simulink model "CM010C_GmG2kcaMcuCfg"  (R2013b)
settings: Solver=FixedStepDiscrete  SolverMode=SingleTasking  StartTime=0.0  StopTime=1  FixedStep=0.0005  RelTol=1e-3
values from neighbouring files (symbols this model uses):
  BATTVLTGSCAGFAC_ULS_F32 = DataDict.Constant    [CM010C_GmG2kcaMcuCfg_DataDict.m]
  BATTVLTGSWD1SCAGFAC_ULS_F32 = DataDict.Constant    [CM010C_GmG2kcaMcuCfg_DataDict.m]
undefined symbols (not defined in the file or in its folder): sigbuilder_block
libraries: CM010C_GmG2kcaMcuCfg_ModelLibrary x48, simulink x32
(part 2 of 2)

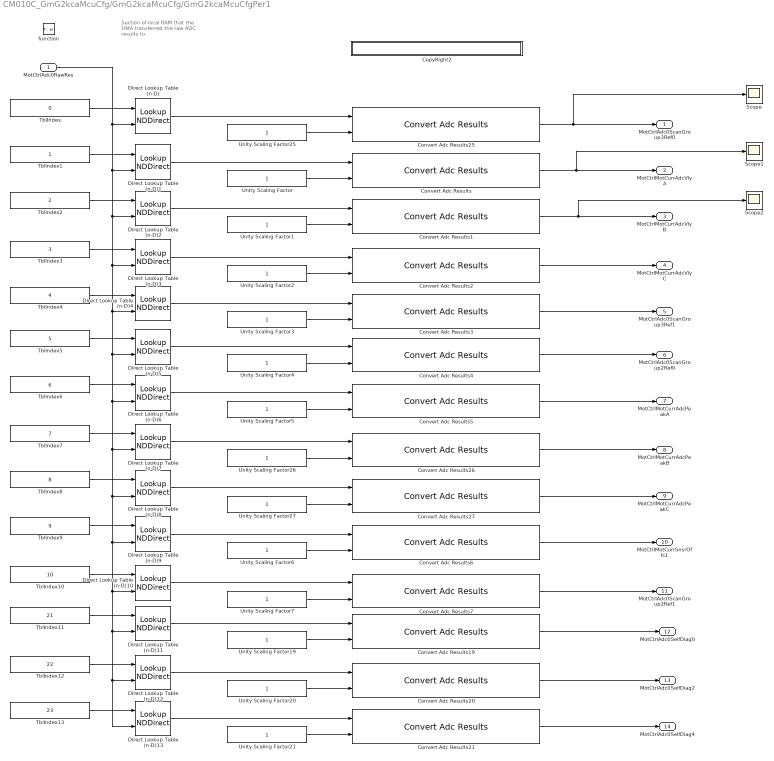
== system CM010C_GmG2kcaMcuCfg/GmG2kcaMcuCfg/GmG2kcaMcuCfgPer1 ==
  note: Section of local RAM that the
      | DMA transferred the raw
      | ADC results to
  MotCtrlAdc0RawRes : Inport
  function : TriggerPort  TriggerType=function-call
  Convert Adc Results{,1..7,19..21,25..27} (14 alike) : CM010C_GmG2kcaMcuCfg_ModelLibrary/Convert Adc Results
  CopyRight2 : Subsystem  Description=|  mask(Copyright Information){none=on}
      | Copyright info block.                                               
      |                                                                     
      | Place copyright information at the top of every subsystem in design.
      mask prompts: none "No parameters"
      mask help: Place copyright information at the top of every subsystem in design.
      mask Display:
      | NxtrConf = 'Nexteer Confidential';
      | 
      | sys = bdroot; %handle for the current model ("system")
      | first = get_param(sys,'Created');
      | first = first(end-3:end);  %year is last four digits
      | 
      | last = get_param(sys,'LastModifiedDate');
      | if isempty(last)
      |     last = datestr(now,'yyyy');
      | else
      |     last = last(end-3:end);
      | end
      | 
      | if strcmp(first,last)
      |     fprintf('%s -- Copyright %s Nexteer',NxtrConf,first)
      | else
      |     fprintf('%s -- %s%s- %s Nexteer',NxtrConf,char(169),first,last)
      | end
  Direct Lookup Table (n-D){,1..13} (14 alike) : LookupNDDirect  NumberOfTableDimensions=1  TableIsInput=on
  Scope : Scope
  Scope1 : Scope
  Scope2 : Scope
      settings: SaveName=ScopeData2
  TblIndex : Constant  Value=0  OutDataTypeStr=Inherit: Inherit via back propagation
  TblIndex1 : Constant  OutDataTypeStr=Inherit: Inherit via back propagation
  TblIndex10 : Constant  Value=10  OutDataTypeStr=Inherit: Inherit via back propagation
  TblIndex11 : Constant  Value=21  OutDataTypeStr=Inherit: Inherit via back propagation
  TblIndex12 : Constant  Value=22  OutDataTypeStr=Inherit: Inherit via back propagation
  TblIndex13 : Constant  Value=23  OutDataTypeStr=Inherit: Inherit via back propagation
  TblIndex2 : Constant  Value=2  OutDataTypeStr=Inherit: Inherit via back propagation
  TblIndex3 : Constant  Value=3  OutDataTypeStr=Inherit: Inherit via back propagation
  TblIndex4 : Constant  Value=4  OutDataTypeStr=Inherit: Inherit via back propagation
  TblIndex5 : Constant  Value=5  OutDataTypeStr=Inherit: Inherit via back propagation
  TblIndex6 : Constant  Value=6  OutDataTypeStr=Inherit: Inherit via back propagation
  TblIndex7 : Constant  Value=7  OutDataTypeStr=Inherit: Inherit via back propagation
  TblIndex8 : Constant  Value=8  OutDataTypeStr=Inherit: Inherit via back propagation
  TblIndex9 : Constant  Value=9  OutDataTypeStr=Inherit: Inherit via back propagation
  Unity Scaling Factor{,1..7,19..21,25..27} (14 alike) : Constant  OutDataTypeStr=single
  MotCtrlAdc0ScanGroup3Ref0 : Outport
  MotCtrlMotCurrAdcVlyA : Outport  Port=2
  MotCtrlMotCurrAdcVlyB : Outport  Port=3
  MotCtrlMotCurrAdcVlyC : Outport  Port=4
  MotCtrlAdc0ScanGroup3Ref1 : Outport  Port=5
  MotCtrlAdc0ScanGroup2Ref0 : Outport  Port=6
  MotCtrlMotCurrAdcPeakA : Outport  Port=7
  MotCtrlMotCurrAdcPeakB : Outport  Port=8
  MotCtrlMotCurrAdcPeakC : Outport  Port=9
  MotCtrlMotCurrSnsrOffs1 : Outport  Port=10
  MotCtrlAdc0ScanGroup2Ref1 : Outport  Port=11
  MotCtrlAdc0SelfDiag0 : Outport  Port=12
  MotCtrlAdc0SelfDiag2 : Outport  Port=13
  MotCtrlAdc0SelfDiag4 : Outport  Port=14
  wires:
  Unity Scaling Factor/1 -> Convert Adc Results/2
  Unity Scaling Factor1/1 -> Convert Adc Results1/2
  Unity Scaling Factor2/1 -> Convert Adc Results2/2
  Unity Scaling Factor3/1 -> Convert Adc Results3/2
  Unity Scaling Factor4/1 -> Convert Adc Results4/2
  Unity Scaling Factor5/1 -> Convert Adc Results5/2
  Unity Scaling Factor6/1 -> Convert Adc Results6/2
  Unity Scaling Factor7/1 -> Convert Adc Results7/2
  Unity Scaling Factor19/1 -> Convert Adc Results19/2
  Unity Scaling Factor20/1 -> Convert Adc Results20/2
  Direct Lookup Table (n-D)/1 -> Convert Adc Results25/1
  Unity Scaling Factor21/1 -> Convert Adc Results21/2
  Convert Adc Results2/1 -> MotCtrlMotCurrAdcVlyC/1
  Convert Adc Results19/1 -> MotCtrlAdc0SelfDiag0/1
  Convert Adc Results20/1 -> MotCtrlAdc0SelfDiag2/1
  Convert Adc Results21/1 -> MotCtrlAdc0SelfDiag4/1
  Unity Scaling Factor25/1 -> Convert Adc Results25/2
  Unity Scaling Factor26/1 -> Convert Adc Results26/2
  Unity Scaling Factor27/1 -> Convert Adc Results27/2
  Convert Adc Results1/1 -> Scope2/1, MotCtrlMotCurrAdcVlyB/1
  Convert Adc Results/1 -> Scope1/1, MotCtrlMotCurrAdcVlyA/1
  Convert Adc Results3/1 -> MotCtrlAdc0ScanGroup3Ref1/1
  Convert Adc Results4/1 -> MotCtrlAdc0ScanGroup2Ref0/1
  Convert Adc Results5/1 -> MotCtrlMotCurrAdcPeakA/1
  Convert Adc Results26/1 -> MotCtrlMotCurrAdcPeakB/1
  Convert Adc Results27/1 -> MotCtrlMotCurrAdcPeakC/1
  Convert Adc Results6/1 -> MotCtrlMotCurrSnsrOffs1/1
  Convert Adc Results7/1 -> MotCtrlAdc0ScanGroup2Ref1/1
  TblIndex/1 -> Direct Lookup Table (n-D)/1
  Convert Adc Results25/1 -> Scope/1, MotCtrlAdc0ScanGroup3Ref0/1
  TblIndex1/1 -> Direct Lookup Table (n-D)1/1
  TblIndex2/1 -> Direct Lookup Table (n-D)2/1
  Direct Lookup Table (n-D)1/1 -> Convert Adc Results/1
  Direct Lookup Table (n-D)2/1 -> Convert Adc Results1/1
  TblIndex3/1 -> Direct Lookup Table (n-D)3/1
  TblIndex4/1 -> Direct Lookup Table (n-D)4/1
  TblIndex5/1 -> Direct Lookup Table (n-D)5/1
  Direct Lookup Table (n-D)3/1 -> Convert Adc Results2/1
  Direct Lookup Table (n-D)4/1 -> Convert Adc Results3/1
  Direct Lookup Table (n-D)5/1 -> Convert Adc Results4/1
  TblIndex6/1 -> Direct Lookup Table (n-D)6/1
  TblIndex7/1 -> Direct Lookup Table (n-D)7/1
  TblIndex8/1 -> Direct Lookup Table (n-D)8/1
  TblIndex9/1 -> Direct Lookup Table (n-D)9/1
  TblIndex10/1 -> Direct Lookup Table (n-D)10/1
  TblIndex11/1 -> Direct Lookup Table (n-D)11/1
  Direct Lookup Table (n-D)6/1 -> Convert Adc Results5/1
  Direct Lookup Table (n-D)7/1 -> Convert Adc Results26/1
  Direct Lookup Table (n-D)8/1 -> Convert Adc Results27/1
  Direct Lookup Table (n-D)9/1 -> Convert Adc Results6/1
  Direct Lookup Table (n-D)10/1 -> Convert Adc Results7/1
  Direct Lookup Table (n-D)11/1 -> Convert Adc Results19/1
  TblIndex12/1 -> Direct Lookup Table (n-D)12/1
  MotCtrlAdc0RawRes/1 -> Direct Lookup Table (n-D)13/2, Direct Lookup Table (n-D)12/2, Direct Lookup Table (n-D)11/2, Direct Lookup Table (n-D)10/2, Direct Lookup Table (n-D)9/2, Direct Lookup Table (n-D)8/2, Direct Lookup Table (n-D)7/2, Direct Lookup Table (n-D)6/2, Direct Lookup Table (n-D)5/2, Direct Lookup Table (n-D)4/2, Direct Lookup Table (n-D)3/2, Direct Lookup Table (n-D)2/2, Direct Lookup Table (n-D)1/2, Direct Lookup Table (n-D)/2
  TblIndex13/1 -> Direct Lookup Table (n-D)13/1
  Direct Lookup Table (n-D)12/1 -> Convert Adc Results20/1
  Direct Lookup Table (n-D)13/1 -> Convert Adc Results21/1

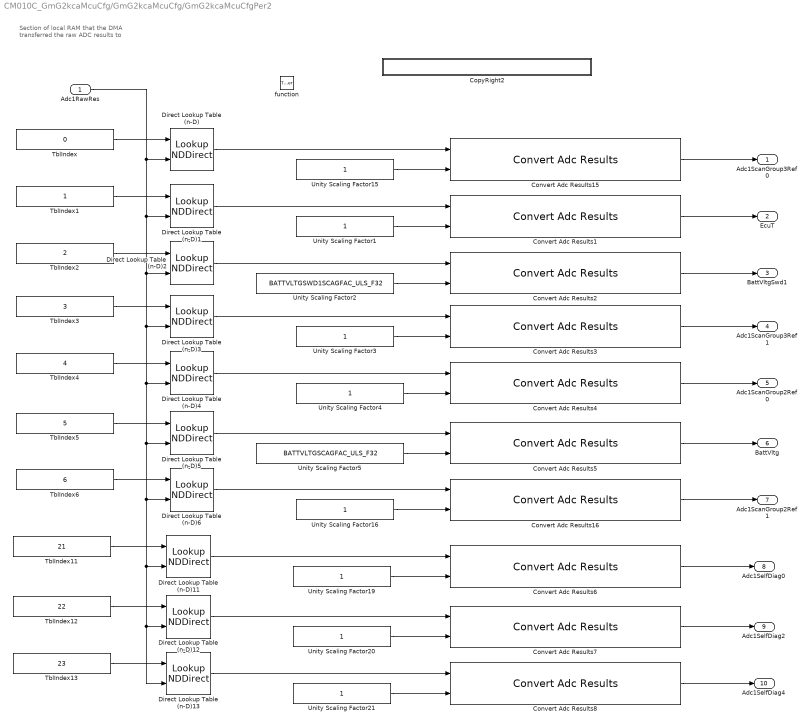
== system CM010C_GmG2kcaMcuCfg/GmG2kcaMcuCfg/GmG2kcaMcuCfgPer2 ==
  note: Section of local RAM that the
      | DMA transferred the raw
      | ADC results to
  Adc1RawRes : Inport
  function : TriggerPort  TriggerType=function-call
  Convert Adc Results{1..8,15..16} (10 alike) : CM010C_GmG2kcaMcuCfg_ModelLibrary/Convert Adc Results
  CopyRight2 : Subsystem  Description=|  mask(Copyright Information){none=on}
      | Copyright info block.                                               
      |                                                                     
      | Place copyright information at the top of every subsystem in design.
      mask prompts: none "No parameters"
      mask help: Place copyright information at the top of every subsystem in design.
      mask Display:
      | NxtrConf = 'Nexteer Confidential';
      | 
      | sys = bdroot; %handle for the current model ("system")
      | first = get_param(sys,'Created');
      | first = first(end-3:end);  %year is last four digits
      | 
      | last = get_param(sys,'LastModifiedDate');
      | if isempty(last)
      |     last = datestr(now,'yyyy');
      | else
      |     last = last(end-3:end);
      | end
      | 
      | if strcmp(first,last)
      |     fprintf('%s -- Copyright %s Nexteer',NxtrConf,first)
      | else
      |     fprintf('%s -- %s%s- %s Nexteer',NxtrConf,char(169),first,last)
      | end
  Direct Lookup Table (n-D){,1..6,11..13} (10 alike) : LookupNDDirect  NumberOfTableDimensions=1  TableIsInput=on
  TblIndex : Constant  Value=0  OutDataTypeStr=Inherit: Inherit via back propagation
  TblIndex1 : Constant  OutDataTypeStr=Inherit: Inherit via back propagation
  TblIndex11 : Constant  Value=21  OutDataTypeStr=Inherit: Inherit via back propagation
  TblIndex12 : Constant  Value=22  OutDataTypeStr=Inherit: Inherit via back propagation
  TblIndex13 : Constant  Value=23  OutDataTypeStr=Inherit: Inherit via back propagation
  TblIndex2 : Constant  Value=2  OutDataTypeStr=Inherit: Inherit via back propagation
  TblIndex3 : Constant  Value=3  OutDataTypeStr=Inherit: Inherit via back propagation
  TblIndex4 : Constant  Value=4  OutDataTypeStr=Inherit: Inherit via back propagation
  TblIndex5 : Constant  Value=5  OutDataTypeStr=Inherit: Inherit via back propagation
  TblIndex6 : Constant  Value=6  OutDataTypeStr=Inherit: Inherit via back propagation
  Unity Scaling Factor{1,3..4,15..16,19..21} (8 alike) : Constant  OutDataTypeStr=single
  Unity Scaling Factor2 : Constant  Value=BATTVLTGSWD1SCAGFAC_ULS_F32  OutDataTypeStr=single
  Unity Scaling Factor5 : Constant  Value=BATTVLTGSCAGFAC_ULS_F32  OutDataTypeStr=single
  Adc1ScanGroup3Ref0 : Outport
  EcuT : Outport  Port=2
  BattVltgSwd1 : Outport  Port=3
  Adc1ScanGroup3Ref1 : Outport  Port=4
  Adc1ScanGroup2Ref0 : Outport  Port=5
  BattVltg : Outport  Port=6
  Adc1ScanGroup2Ref1 : Outport  Port=7
  Adc1SelfDiag0 : Outport  Port=8
  Adc1SelfDiag2 : Outport  Port=9
  Adc1SelfDiag4 : Outport  Port=10
  wires:
  Convert Adc Results8/1 -> Adc1SelfDiag4/1
  Convert Adc Results7/1 -> Adc1SelfDiag2/1
  Convert Adc Results6/1 -> Adc1SelfDiag0/1
  Convert Adc Results1/1 -> EcuT/1
  Unity Scaling Factor21/1 -> Convert Adc Results8/2
  Direct Lookup Table (n-D)13/1 -> Convert Adc Results8/1
  Unity Scaling Factor20/1 -> Convert Adc Results7/2
  Direct Lookup Table (n-D)12/1 -> Convert Adc Results7/1
  Unity Scaling Factor19/1 -> Convert Adc Results6/2
  Direct Lookup Table (n-D)11/1 -> Convert Adc Results6/1
  Unity Scaling Factor5/1 -> Convert Adc Results5/2
  Unity Scaling Factor4/1 -> Convert Adc Results4/2
  Unity Scaling Factor3/1 -> Convert Adc Results3/2
  Unity Scaling Factor2/1 -> Convert Adc Results2/2
  Unity Scaling Factor1/1 -> Convert Adc Results1/2
  Unity Scaling Factor15/1 -> Convert Adc Results15/2
  Convert Adc Results15/1 -> Adc1ScanGroup3Ref0/1
  Unity Scaling Factor16/1 -> Convert Adc Results16/2
  Direct Lookup Table (n-D)/1 -> Convert Adc Results15/1
  Direct Lookup Table (n-D)1/1 -> Convert Adc Results1/1
  Direct Lookup Table (n-D)2/1 -> Convert Adc Results2/1
  Direct Lookup Table (n-D)3/1 -> Convert Adc Results3/1
  Direct Lookup Table (n-D)4/1 -> Convert Adc Results4/1
  Direct Lookup Table (n-D)5/1 -> Convert Adc Results5/1
  Direct Lookup Table (n-D)6/1 -> Convert Adc Results16/1
  Convert Adc Results2/1 -> BattVltgSwd1/1
  Convert Adc Results3/1 -> Adc1ScanGroup3Ref1/1
  Convert Adc Results4/1 -> Adc1ScanGroup2Ref0/1
  Convert Adc Results5/1 -> BattVltg/1
  Convert Adc Results16/1 -> Adc1ScanGroup2Ref1/1
  TblIndex/1 -> Direct Lookup Table (n-D)/1
  TblIndex1/1 -> Direct Lookup Table (n-D)1/1
  TblIndex2/1 -> Direct Lookup Table (n-D)2/1
  TblIndex3/1 -> Direct Lookup Table (n-D)3/1
  TblIndex4/1 -> Direct Lookup Table (n-D)4/1
  TblIndex5/1 -> Direct Lookup Table (n-D)5/1
  TblIndex6/1 -> Direct Lookup Table (n-D)6/1
  TblIndex11/1 -> Direct Lookup Table (n-D)11/1
  TblIndex12/1 -> Direct Lookup Table (n-D)12/1
  Adc1RawRes/1 -> Direct Lookup Table (n-D)/2, Direct Lookup Table (n-D)1/2, Direct Lookup Table (n-D)2/2, Direct Lookup Table (n-D)3/2, Direct Lookup Table (n-D)4/2, Direct Lookup Table (n-D)5/2, Direct Lookup Table (n-D)6/2, Direct Lookup Table (n-D)11/2, Direct Lookup Table (n-D)12/2, Direct Lookup Table (n-D)13/2
  TblIndex13/1 -> Direct Lookup Table (n-D)13/1

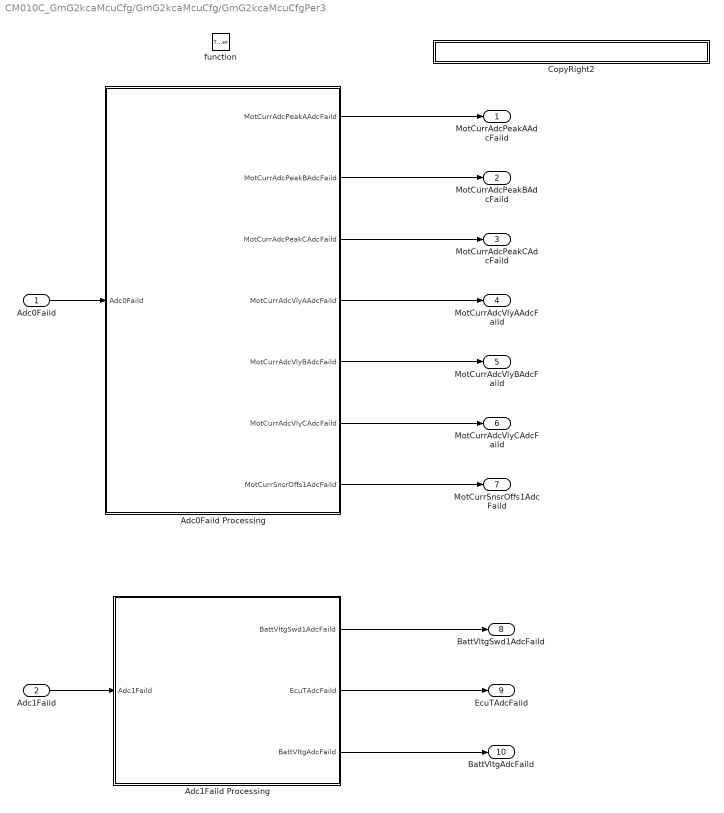
== system CM010C_GmG2kcaMcuCfg/GmG2kcaMcuCfg/GmG2kcaMcuCfgPer3 ==
  Adc0Faild : Inport
  Adc1Faild : Inport  Port=2
  function : TriggerPort  TriggerType=function-call
  Adc0Faild Processing : Subsystem  TreatAsAtomicUnit=on
  Adc1Faild Processing : Subsystem  TreatAsAtomicUnit=on
  CopyRight2 : Subsystem  Description=|  mask(Copyright Information){none=on}
      | Copyright info block.                                               
      |                                                                     
      | Place copyright information at the top of every subsystem in design.
      mask prompts: none "No parameters"
      mask help: Place copyright information at the top of every subsystem in design.
      mask Display:
      | NxtrConf = 'Nexteer Confidential';
      | 
      | sys = bdroot; %handle for the current model ("system")
      | first = get_param(sys,'Created');
      | first = first(end-3:end);  %year is last four digits
      | 
      | last = get_param(sys,'LastModifiedDate');
      | if isempty(last)
      |     last = datestr(now,'yyyy');
      | else
      |     last = last(end-3:end);
      | end
      | 
      | if strcmp(first,last)
      |     fprintf('%s -- Copyright %s Nexteer',NxtrConf,first)
      | else
      |     fprintf('%s -- %s%s- %s Nexteer',NxtrConf,char(169),first,last)
      | end
  MotCurrAdcPeakAAdcFaild : Outport
  MotCurrAdcPeakBAdcFaild : Outport  Port=2
  MotCurrAdcPeakCAdcFaild : Outport  Port=3
  MotCurrAdcVlyAAdcFaild : Outport  Port=4
  MotCurrAdcVlyBAdcFaild : Outport  Port=5
  MotCurrAdcVlyCAdcFaild : Outport  Port=6
  MotCurrSnsrOffs1AdcFaild : Outport  Port=7
  BattVltgSwd1AdcFaild : Outport  Port=8
  EcuTAdcFaild : Outport  Port=9
  BattVltgAdcFaild : Outport  Port=10
  wires:
  Adc0Faild/1 -> Adc0Faild Processing/1(Adc0Faild)
  Adc0Faild Processing/1(MotCurrAdcPeakAAdcFaild) -> MotCurrAdcPeakAAdcFaild/1
  Adc0Faild Processing/2(MotCurrAdcPeakBAdcFaild) -> MotCurrAdcPeakBAdcFaild/1
  Adc0Faild Processing/3(MotCurrAdcPeakCAdcFaild) -> MotCurrAdcPeakCAdcFaild/1
  Adc0Faild Processing/4(MotCurrAdcVlyAAdcFaild) -> MotCurrAdcVlyAAdcFaild/1
  Adc0Faild Processing/5(MotCurrAdcVlyBAdcFaild) -> MotCurrAdcVlyBAdcFaild/1
  Adc0Faild Processing/6(MotCurrAdcVlyCAdcFaild) -> MotCurrAdcVlyCAdcFaild/1
  Adc0Faild Processing/7(MotCurrSnsrOffs1AdcFaild) -> MotCurrSnsrOffs1AdcFaild/1
  Adc1Faild/1 -> Adc1Faild Processing/1(Adc1Faild)
  Adc1Faild Processing/1(BattVltgSwd1AdcFaild) -> BattVltgSwd1AdcFaild/1
  Adc1Faild Processing/2(EcuTAdcFaild) -> EcuTAdcFaild/1
  Adc1Faild Processing/3(BattVltgAdcFaild) -> BattVltgAdcFaild/1

== system CM010C_GmG2kcaMcuCfg/GmG2kcaMcuCfg/GmG2kcaMcuCfgInit1/CopyRight2 ==

== system CM010C_GmG2kcaMcuCfg/GmG2kcaMcuCfg/GmG2kcaMcuCfgInit1/Register Initialization ==
  note: GmG2kcaMcuCfg Configuration
      | Initialize the PIC2B registers from the following sources in the order listed:
      |
      |
      | 1. Run Adc0CfgAndUseInit1 - this means to run the AdcCfgInit function first before this init function, there is no client or server call
      | 2  Run Adc1CfgAndUseInit1 - this means to run the AdcCfgInit function first before this init function, there is no client or server call
      | 3. CM010C_GmG2kcaMcuCfg_RegisterConfiguration.xlsm
      |     Order by row
  CopyRight2 : Subsystem  Description=|  mask(Copyright Information){none=on}
      | Copyright info block.                                               
      |                                                                     
      | Place copyright information at the top of every subsystem in design.
      mask prompts: none "No parameters"
      mask help: Place copyright information at the top of every subsystem in design.
      mask Display:
      | NxtrConf = 'Nexteer Confidential';
      | 
      | sys = bdroot; %handle for the current model ("system")
      | first = get_param(sys,'Created');
      | first = first(end-3:end);  %year is last four digits
      | 
      | last = get_param(sys,'LastModifiedDate');
      | if isempty(last)
      |     last = datestr(now,'yyyy');
      | else
      |     last = last(end-3:end);
      | end
      | 
      | if strcmp(first,last)
      |     fprintf('%s -- Copyright %s Nexteer',NxtrConf,first)
      | else
      |     fprintf('%s -- %s%s- %s Nexteer',NxtrConf,char(169),first,last)
      | end

== system CM010C_GmG2kcaMcuCfg/GmG2kcaMcuCfg/GmG2kcaMcuCfgInit2/CopyRight2 ==

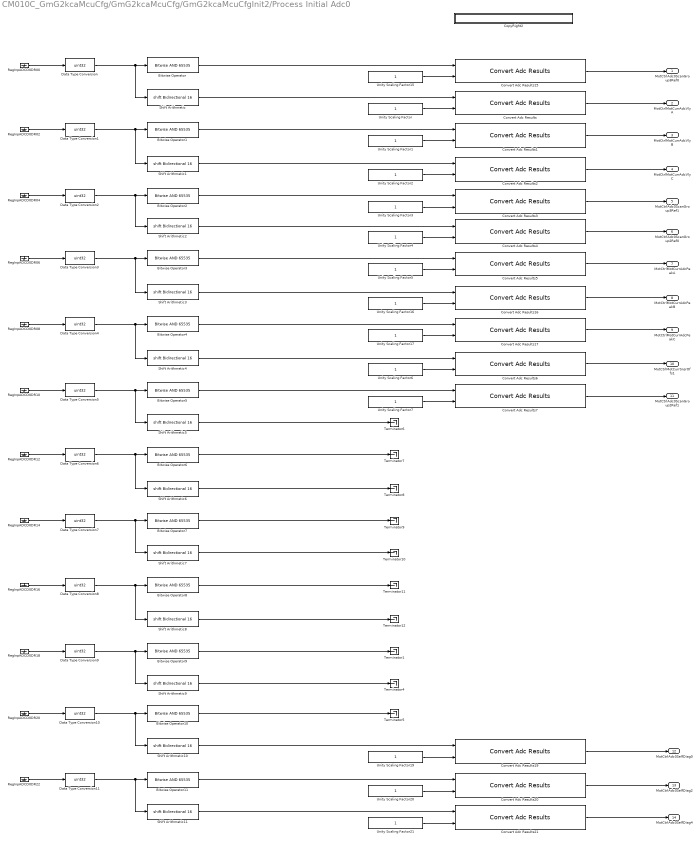
== system CM010C_GmG2kcaMcuCfg/GmG2kcaMcuCfg/GmG2kcaMcuCfgInit2/Process Initial Adc0 ==
  Bitwise Operator{,1..11} (12 alike) : simulink/Logic and Bit Operations/Bitwise Operator  logicop=AND  UseBitMask=on  BitMask=65535  BitMaskRealWorld=Stored Integer
  Convert Adc Results{,1..7,15..17,19..21} (14 alike) : CM010C_GmG2kcaMcuCfg_ModelLibrary/Convert Adc Results
  CopyRight2 : Subsystem  Description=|  mask(Copyright Information){none=on}
      | Copyright info block.                                               
      |                                                                     
      | Place copyright information at the top of every subsystem in design.
      mask prompts: none "No parameters"
      mask help: Place copyright information at the top of every subsystem in design.
      mask Display:
      | NxtrConf = 'Nexteer Confidential';
      | 
      | sys = bdroot; %handle for the current model ("system")
      | first = get_param(sys,'Created');
      | first = first(end-3:end);  %year is last four digits
      | 
      | last = get_param(sys,'LastModifiedDate');
      | if isempty(last)
      |     last = datestr(now,'yyyy');
      | else
      |     last = last(end-3:end);
      | end
      | 
      | if strcmp(first,last)
      |     fprintf('%s -- Copyright %s Nexteer',NxtrConf,first)
      | else
      |     fprintf('%s -- %s%s- %s Nexteer',NxtrConf,char(169),first,last)
      | end
  Data Type Conversion{,1..11} (12 alike) : DataTypeConversion  OutDataTypeStr=uint32
  RegInpADCD0DR00 : Ground
  RegInpADCD0DR02 : Ground
  RegInpADCD0DR04 : Ground
  RegInpADCD0DR06 : Ground
  RegInpADCD0DR08 : Ground
  RegInpADCD0DR{10,12,14,16,18,20,22} (7 alike) : Ground
  Shift Arithmetic{,1..11} (12 alike) : ArithShift  BitShiftNumber=16
  Terminator{1,4..12} (10 alike) : Terminator
  Unity Scaling Factor{,1..7,15..17,19..21} (14 alike) : Constant  OutDataTypeStr=single
  MotCtrlAdc0ScanGroup3Ref0 : Outport
  MotCtrlMotCurrAdcVlyA : Outport  Port=2
  MotCtrlMotCurrAdcVlyB : Outport  Port=3
  MotCtrlMotCurrAdcVlyC : Outport  Port=4
  MotCtrlAdc0ScanGroup3Ref1 : Outport  Port=5
  MotCtrlAdc0ScanGroup2Ref0 : Outport  Port=6
  MotCtrlMotCurrAdcPeakA : Outport  Port=7
  MotCtrlMotCurrAdcPeakB : Outport  Port=8
  MotCtrlMotCurrAdcPeakC : Outport  Port=9
  MotCtrlMotCurrSnsrOffs1 : Outport  Port=10
  MotCtrlAdc0ScanGroup2Ref1 : Outport  Port=11
  MotCtrlAdc0SelfDiag0 : Outport  Port=12
  MotCtrlAdc0SelfDiag2 : Outport  Port=13
  MotCtrlAdc0SelfDiag4 : Outport  Port=14
  wires:
  Unity Scaling Factor/1 -> Convert Adc Results/2
  Unity Scaling Factor1/1 -> Convert Adc Results1/2
  Unity Scaling Factor2/1 -> Convert Adc Results2/2
  Unity Scaling Factor3/1 -> Convert Adc Results3/2
  Unity Scaling Factor4/1 -> Convert Adc Results4/2
  Unity Scaling Factor5/1 -> Convert Adc Results5/2
  Unity Scaling Factor19/1 -> Convert Adc Results19/2
  Unity Scaling Factor20/1 -> Convert Adc Results20/2
  Unity Scaling Factor21/1 -> Convert Adc Results21/2
  Convert Adc Results/1 -> MotCtrlMotCurrAdcVlyA/1
  Convert Adc Results1/1 -> MotCtrlMotCurrAdcVlyB/1
  Convert Adc Results2/1 -> MotCtrlMotCurrAdcVlyC/1
  Convert Adc Results19/1 -> MotCtrlAdc0SelfDiag0/1
  Convert Adc Results20/1 -> MotCtrlAdc0SelfDiag2/1
  Convert Adc Results21/1 -> MotCtrlAdc0SelfDiag4/1
  RegInpADCD0DR00/1 -> Data Type Conversion/1
  RegInpADCD0DR02/1 -> Data Type Conversion1/1
  RegInpADCD0DR04/1 -> Data Type Conversion2/1
  RegInpADCD0DR06/1 -> Data Type Conversion3/1
  RegInpADCD0DR08/1 -> Data Type Conversion4/1
  RegInpADCD0DR10/1 -> Data Type Conversion5/1
  RegInpADCD0DR12/1 -> Data Type Conversion6/1
  RegInpADCD0DR14/1 -> Data Type Conversion7/1
  RegInpADCD0DR16/1 -> Data Type Conversion8/1
  RegInpADCD0DR18/1 -> Data Type Conversion9/1
  RegInpADCD0DR20/1 -> Data Type Conversion10/1
  RegInpADCD0DR22/1 -> Data Type Conversion11/1
  Shift Arithmetic11/1 -> Convert Adc Results21/1
  Bitwise Operator11/1 -> Convert Adc Results20/1
  Shift Arithmetic10/1 -> Convert Adc Results19/1
  Bitwise Operator10/1 -> Terminator5/1
  Shift Arithmetic9/1 -> Terminator4/1
  Unity Scaling Factor15/1 -> Convert Adc Results15/2
  Convert Adc Results15/1 -> MotCtrlAdc0ScanGroup3Ref0/1
  Bitwise Operator/1 -> Convert Adc Results15/1
  Shift Arithmetic/1 -> Convert Adc Results/1
  Bitwise Operator1/1 -> Convert Adc Results1/1
  Shift Arithmetic1/1 -> Convert Adc Results2/1
  Bitwise Operator2/1 -> Convert Adc Results3/1
  Shift Arithmetic2/1 -> Convert Adc Results4/1
  Bitwise Operator3/1 -> Convert Adc Results5/1
  Unity Scaling Factor16/1 -> Convert Adc Results16/2
  Shift Arithmetic3/1 -> Convert Adc Results16/1
  Unity Scaling Factor17/1 -> Convert Adc Results17/2
  Bitwise Operator4/1 -> Convert Adc Results17/1
  Bitwise Operator9/1 -> Terminator1/1
  Convert Adc Results3/1 -> MotCtrlAdc0ScanGroup3Ref1/1
  Convert Adc Results4/1 -> MotCtrlAdc0ScanGroup2Ref0/1
  Convert Adc Results5/1 -> MotCtrlMotCurrAdcPeakA/1
  Convert Adc Results16/1 -> MotCtrlMotCurrAdcPeakB/1
  Convert Adc Results17/1 -> MotCtrlMotCurrAdcPeakC/1
  Shift Arithmetic5/1 -> Terminator6/1
  Bitwise Operator7/1 -> Terminator9/1
  Shift Arithmetic6/1 -> Terminator8/1
  Bitwise Operator6/1 -> Terminator7/1
  Shift Arithmetic8/1 -> Terminator12/1
  Bitwise Operator8/1 -> Terminator11/1
  Shift Arithmetic7/1 -> Terminator10/1
  Unity Scaling Factor6/1 -> Convert Adc Results6/2
  Shift Arithmetic4/1 -> Convert Adc Results6/1
  Unity Scaling Factor7/1 -> Convert Adc Results7/2
  Bitwise Operator5/1 -> Convert Adc Results7/1
  Convert Adc Results6/1 -> MotCtrlMotCurrSnsrOffs1/1
  Convert Adc Results7/1 -> MotCtrlAdc0ScanGroup2Ref1/1
  Data Type Conversion/1 -> Bitwise Operator/1, Shift Arithmetic/1
  Data Type Conversion1/1 -> Shift Arithmetic1/1, Bitwise Operator1/1
  Data Type Conversion2/1 -> Bitwise Operator2/1, Shift Arithmetic2/1
  Data Type Conversion3/1 -> Shift Arithmetic3/1, Bitwise Operator3/1
  Data Type Conversion4/1 -> Bitwise Operator4/1, Shift Arithmetic4/1
  Data Type Conversion5/1 -> Bitwise Operator5/1, Shift Arithmetic5/1
  Data Type Conversion6/1 -> Bitwise Operator6/1, Shift Arithmetic6/1
  Data Type Conversion7/1 -> Bitwise Operator7/1, Shift Arithmetic7/1
  Data Type Conversion8/1 -> Bitwise Operator8/1, Shift Arithmetic8/1
  Data Type Conversion9/1 -> Bitwise Operator9/1, Shift Arithmetic9/1
  Data Type Conversion10/1 -> Bitwise Operator10/1, Shift Arithmetic10/1
  Data Type Conversion11/1 -> Bitwise Operator11/1, Shift Arithmetic11/1

== system CM010C_GmG2kcaMcuCfg/GmG2kcaMcuCfg/GmG2kcaMcuCfgInit2/Wait for ADC Conversion to Complete ==
  note: Use the following client calls to perform a 25uSec wait.
  CopyRight2 : Subsystem  Description=|  mask(Copyright Information){none=on}
      | Copyright info block.                                               
      |                                                                     
      | Place copyright information at the top of every subsystem in design.
      mask prompts: none "No parameters"
      mask help: Place copyright information at the top of every subsystem in design.
      mask Display:
      | NxtrConf = 'Nexteer Confidential';
      | 
      | sys = bdroot; %handle for the current model ("system")
      | first = get_param(sys,'Created');
      | first = first(end-3:end);  %year is last four digits
      | 
      | last = get_param(sys,'LastModifiedDate');
      | if isempty(last)
      |     last = datestr(now,'yyyy');
      | else
      |     last = last(end-3:end);
      | end
      | 
      | if strcmp(first,last)
      |     fprintf('%s -- Copyright %s Nexteer',NxtrConf,first)
      | else
      |     fprintf('%s -- %s%s- %s Nexteer',NxtrConf,char(169),first,last)
      | end
  GetRefTmr1MicroSec32bit : Subsystem  TreatAsAtomicUnit=on
  GetTiSpan1MicroSec32bit : Subsystem  TreatAsAtomicUnit=on
  Ground : Ground
  Terminator : Terminator
  Terminator1 : Terminator
  wires:
  GetRefTmr1MicroSec32bit/1(RefTmr) -> Terminator/1
  GetTiSpan1MicroSec32bit/1(TiSpan) -> Terminator1/1
  Ground/1 -> GetTiSpan1MicroSec32bit/1(RefTmr)

== system CM010C_GmG2kcaMcuCfg/GmG2kcaMcuCfg/GmG2kcaMcuCfgInit3/CopyRight2 ==

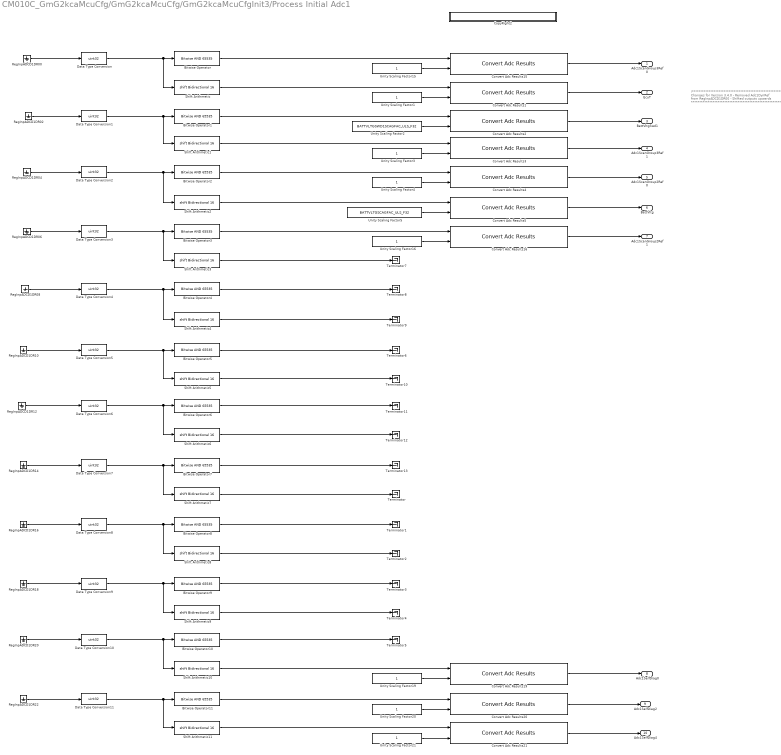
== system CM010C_GmG2kcaMcuCfg/GmG2kcaMcuCfg/GmG2kcaMcuCfgInit3/Process Initial Adc1 ==
  note: /******************************************************
      | Changes for Version 3.4.0
      | - Removed Adc1DynRef from RegInpADCD1DR00
      | - Shifted outputs upwards
      | ******************************************************/
  Bitwise Operator{,1..11} (12 alike) : simulink/Logic and Bit Operations/Bitwise Operator  logicop=AND  UseBitMask=on  BitMask=65535  BitMaskRealWorld=Stored Integer
  Convert Adc Results{1..5,15..16,19..21} (10 alike) : CM010C_GmG2kcaMcuCfg_ModelLibrary/Convert Adc Results
  CopyRight2 : Subsystem  Description=|  mask(Copyright Information){none=on}
      | Copyright info block.                                               
      |                                                                     
      | Place copyright information at the top of every subsystem in design.
      mask prompts: none "No parameters"
      mask help: Place copyright information at the top of every subsystem in design.
      mask Display:
      | NxtrConf = 'Nexteer Confidential';
      | 
      | sys = bdroot; %handle for the current model ("system")
      | first = get_param(sys,'Created');
      | first = first(end-3:end);  %year is last four digits
      | 
      | last = get_param(sys,'LastModifiedDate');
      | if isempty(last)
      |     last = datestr(now,'yyyy');
      | else
      |     last = last(end-3:end);
      | end
      | 
      | if strcmp(first,last)
      |     fprintf('%s -- Copyright %s Nexteer',NxtrConf,first)
      | else
      |     fprintf('%s -- %s%s- %s Nexteer',NxtrConf,char(169),first,last)
      | end
  Data Type Conversion{,1..11} (12 alike) : DataTypeConversion  OutDataTypeStr=uint32
  RegInpADCD1DR00 : Ground
  RegInpADCD1DR02 : Ground
  RegInpADCD1DR04 : Ground
  RegInpADCD1DR06 : Ground
  RegInpADCD1DR08 : Ground
  RegInpADCD1DR{10,12,14,16,18,20,22} (7 alike) : Ground
  Shift Arithmetic{,1..11} (12 alike) : ArithShift  BitShiftNumber=16
  Terminator{,1..13} (14 alike) : Terminator
  Unity Scaling Factor{1,3..4,15..16,19..21} (8 alike) : Constant  OutDataTypeStr=single
  Unity Scaling Factor2 : Constant  Value=BATTVLTGSWD1SCAGFAC_ULS_F32  OutDataTypeStr=single
  Unity Scaling Factor5 : Constant  Value=BATTVLTGSCAGFAC_ULS_F32  OutDataTypeStr=single
  Adc1ScanGroup3Ref0 : Outport
  EcuT : Outport  Port=2
  BattVltgSwd1 : Outport  Port=3
  Adc1ScanGroup3Ref1 : Outport  Port=4
  Adc1ScanGroup2Ref0 : Outport  Port=5
  BattVltg : Outport  Port=6
  Adc1ScanGroup2Ref1 : Outport  Port=7
  Adc1SelfDiag0 : Outport  Port=8
  Adc1SelfDiag2 : Outport  Port=9
  Adc1SelfDiag4 : Outport  Port=10
  wires:
  Convert Adc Results21/1 -> Adc1SelfDiag4/1
  Convert Adc Results20/1 -> Adc1SelfDiag2/1
  Convert Adc Results19/1 -> Adc1SelfDiag0/1
  Convert Adc Results1/1 -> EcuT/1
  Unity Scaling Factor21/1 -> Convert Adc Results21/2
  Unity Scaling Factor20/1 -> Convert Adc Results20/2
  Unity Scaling Factor19/1 -> Convert Adc Results19/2
  Unity Scaling Factor5/1 -> Convert Adc Results5/2
  Unity Scaling Factor4/1 -> Convert Adc Results4/2
  Unity Scaling Factor3/1 -> Convert Adc Results3/2
  Unity Scaling Factor2/1 -> Convert Adc Results2/2
  Unity Scaling Factor1/1 -> Convert Adc Results1/2
  RegInpADCD1DR00/1 -> Data Type Conversion/1
  RegInpADCD1DR02/1 -> Data Type Conversion1/1
  RegInpADCD1DR04/1 -> Data Type Conversion2/1
  RegInpADCD1DR06/1 -> Data Type Conversion3/1
  RegInpADCD1DR08/1 -> Data Type Conversion4/1
  RegInpADCD1DR10/1 -> Data Type Conversion5/1
  RegInpADCD1DR12/1 -> Data Type Conversion6/1
  RegInpADCD1DR14/1 -> Data Type Conversion7/1
  RegInpADCD1DR16/1 -> Data Type Conversion8/1
  RegInpADCD1DR18/1 -> Data Type Conversion9/1
  RegInpADCD1DR20/1 -> Data Type Conversion10/1
  RegInpADCD1DR22/1 -> Data Type Conversion11/1
  Shift Arithmetic11/1 -> Convert Adc Results21/1
  Bitwise Operator11/1 -> Convert Adc Results20/1
  Shift Arithmetic10/1 -> Convert Adc Results19/1
  Bitwise Operator10/1 -> Terminator5/1
  Bitwise Operator9/1 -> Terminator3/1
  Shift Arithmetic9/1 -> Terminator4/1
  Bitwise Operator8/1 -> Terminator1/1
  Shift Arithmetic8/1 -> Terminator2/1
  Shift Arithmetic7/1 -> Terminator/1
  Shift Arithmetic5/1 -> Terminator10/1
  Bitwise Operator6/1 -> Terminator11/1
  Shift Arithmetic6/1 -> Terminator12/1
  Bitwise Operator7/1 -> Terminator13/1
  Unity Scaling Factor15/1 -> Convert Adc Results15/2
  Convert Adc Results15/1 -> Adc1ScanGroup3Ref0/1
  Unity Scaling Factor16/1 -> Convert Adc Results16/2
  Bitwise Operator/1 -> Convert Adc Results15/1
  Shift Arithmetic/1 -> Convert Adc Results1/1
  Bitwise Operator1/1 -> Convert Adc Results2/1
  Shift Arithmetic1/1 -> Convert Adc Results3/1
  Bitwise Operator2/1 -> Convert Adc Results4/1
  Shift Arithmetic2/1 -> Convert Adc Results5/1
  Bitwise Operator3/1 -> Convert Adc Results16/1
  Bitwise Operator5/1 -> Terminator6/1
  Convert Adc Results2/1 -> BattVltgSwd1/1
  Convert Adc Results3/1 -> Adc1ScanGroup3Ref1/1
  Convert Adc Results4/1 -> Adc1ScanGroup2Ref0/1
  Convert Adc Results5/1 -> BattVltg/1
  Convert Adc Results16/1 -> Adc1ScanGroup2Ref1/1
  Shift Arithmetic3/1 -> Terminator7/1
  Bitwise Operator4/1 -> Terminator8/1
  Shift Arithmetic4/1 -> Terminator9/1
  Data Type Conversion/1 -> Bitwise Operator/1, Shift Arithmetic/1
  Data Type Conversion1/1 -> Bitwise Operator1/1, Shift Arithmetic1/1
  Data Type Conversion2/1 -> Bitwise Operator2/1, Shift Arithmetic2/1
  Data Type Conversion3/1 -> Bitwise Operator3/1, Shift Arithmetic3/1
  Data Type Conversion4/1 -> Bitwise Operator4/1, Shift Arithmetic4/1
  Data Type Conversion5/1 -> Bitwise Operator5/1, Shift Arithmetic5/1
  Data Type Conversion6/1 -> Bitwise Operator6/1, Shift Arithmetic6/1
  Data Type Conversion7/1 -> Bitwise Operator7/1, Shift Arithmetic7/1
  Data Type Conversion8/1 -> Shift Arithmetic8/1, Bitwise Operator8/1
  Data Type Conversion9/1 -> Bitwise Operator9/1, Shift Arithmetic9/1
  Data Type Conversion10/1 -> Bitwise Operator10/1, Shift Arithmetic10/1
  Data Type Conversion11/1 -> Bitwise Operator11/1, Shift Arithmetic11/1

== system CM010C_GmG2kcaMcuCfg/GmG2kcaMcuCfg/GmG2kcaMcuCfgPer1/CopyRight2 ==

== system CM010C_GmG2kcaMcuCfg/GmG2kcaMcuCfg/GmG2kcaMcuCfgPer2/CopyRight2 ==

== system CM010C_GmG2kcaMcuCfg/GmG2kcaMcuCfg/GmG2kcaMcuCfgPer3/Adc0Faild Processing ==
  Adc0Faild : Inport
  CopyRight2 : Subsystem  Description=|  mask(Copyright Information){none=on}
      | Copyright info block.                                               
      |                                                                     
      | Place copyright information at the top of every subsystem in design.
      mask prompts: none "No parameters"
      mask help: Place copyright information at the top of every subsystem in design.
      mask Display:
      | NxtrConf = 'Nexteer Confidential';
      | 
      | sys = bdroot; %handle for the current model ("system")
      | first = get_param(sys,'Created');
      | first = first(end-3:end);  %year is last four digits
      | 
      | last = get_param(sys,'LastModifiedDate');
      | if isempty(last)
      |     last = datestr(now,'yyyy');
      | else
      |     last = last(end-3:end);
      | end
      | 
      | if strcmp(first,last)
      |     fprintf('%s -- Copyright %s Nexteer',NxtrConf,first)
      | else
      |     fprintf('%s -- %s%s- %s Nexteer',NxtrConf,char(169),first,last)
      | end
  MotCurrAdcPeakAAdcFaild : Outport
  MotCurrAdcPeakBAdcFaild : Outport  Port=2
  MotCurrAdcPeakCAdcFaild : Outport  Port=3
  MotCurrAdcVlyAAdcFaild : Outport  Port=4
  MotCurrAdcVlyBAdcFaild : Outport  Port=5
  MotCurrAdcVlyCAdcFaild : Outport  Port=6
  MotCurrSnsrOffs1AdcFaild : Outport  Port=7
  wires:
  Adc0Faild/1 -> MotCurrSnsrOffs1AdcFaild/1, MotCurrAdcVlyCAdcFaild/1, MotCurrAdcVlyBAdcFaild/1, MotCurrAdcVlyAAdcFaild/1, MotCurrAdcPeakCAdcFaild/1, MotCurrAdcPeakBAdcFaild/1, MotCurrAdcPeakAAdcFaild/1

== system CM010C_GmG2kcaMcuCfg/GmG2kcaMcuCfg/GmG2kcaMcuCfgPer3/Adc1Faild Processing ==
  Adc1Faild : Inport
  CopyRight2 : Subsystem  Description=|  mask(Copyright Information){none=on}
      | Copyright info block.                                               
      |                                                                     
      | Place copyright information at the top of every subsystem in design.
      mask prompts: none "No parameters"
      mask help: Place copyright information at the top of every subsystem in design.
      mask Display:
      | NxtrConf = 'Nexteer Confidential';
      | 
      | sys = bdroot; %handle for the current model ("system")
      | first = get_param(sys,'Created');
      | first = first(end-3:end);  %year is last four digits
      | 
      | last = get_param(sys,'LastModifiedDate');
      | if isempty(last)
      |     last = datestr(now,'yyyy');
      | else
      |     last = last(end-3:end);
      | end
      | 
      | if strcmp(first,last)
      |     fprintf('%s -- Copyright %s Nexteer',NxtrConf,first)
      | else
      |     fprintf('%s -- %s%s- %s Nexteer',NxtrConf,char(169),first,last)
      | end
  BattVltgSwd1AdcFaild : Outport
  EcuTAdcFaild : Outport  Port=2
  BattVltgAdcFaild : Outport  Port=3
  wires:
  Adc1Faild/1 -> BattVltgAdcFaild/1, EcuTAdcFaild/1, BattVltgSwd1AdcFaild/1

== system CM010C_GmG2kcaMcuCfg/GmG2kcaMcuCfg/GmG2kcaMcuCfgPer3/CopyRight2 ==

== system CM010C_GmG2kcaMcuCfg/GmG2kcaMcuCfg/GmG2kcaMcuCfgInit1/Register Initialization/CopyRight2 ==

== system CM010C_GmG2kcaMcuCfg/GmG2kcaMcuCfg/GmG2kcaMcuCfgInit2/Process Initial Adc0/CopyRight2 ==

== system CM010C_GmG2kcaMcuCfg/GmG2kcaMcuCfg/GmG2kcaMcuCfgInit2/Wait for ADC Conversion to Complete/CopyRight2 ==

== system CM010C_GmG2kcaMcuCfg/GmG2kcaMcuCfg/GmG2kcaMcuCfgInit2/Wait for ADC Conversion to Complete/GetRefTmr1MicroSec32bit ==
  Ground : Ground
  RefTmr : Outport
  wires:
  Ground/1 -> RefTmr/1

== system CM010C_GmG2kcaMcuCfg/GmG2kcaMcuCfg/GmG2kcaMcuCfgInit2/Wait for ADC Conversion to Complete/GetTiSpan1MicroSec32bit ==
  RefTmr : Inport
  Ground : Ground
  Terminator : Terminator
  TiSpan : Outport
  wires:
  Ground/1 -> TiSpan/1
  RefTmr/1 -> Terminator/1

== system CM010C_GmG2kcaMcuCfg/GmG2kcaMcuCfg/GmG2kcaMcuCfgInit3/Process Initial Adc1/CopyRight2 ==

== system CM010C_GmG2kcaMcuCfg/GmG2kcaMcuCfg/GmG2kcaMcuCfgPer3/Adc0Faild Processing/CopyRight2 ==

== system CM010C_GmG2kcaMcuCfg/GmG2kcaMcuCfg/GmG2kcaMcuCfgPer3/Adc1Faild Processing/CopyRight2 ==
